simulink model "px4demo_rgbled"  (R2014b)
settings: Solver=ode3  SolverMode=SingleTasking  StartTime=0.0  StopTime=10.0  FixedStep=1/250  RelTol=1e-3
PostLoadFcn:
  | Ts = 1/250;
undefined symbols (not defined in the file): RGBLED_COLOR_ENUM, RGBLED_MODE_ENUM
libraries: pixhawk_sllib x1
settings Model: Creator=skuznick  LastModifiedBy=skuznick
settings OptimizationCC: InlineParams=on  OptimizeModelRefInitCode=on  LifeSpan=1  MaxStackSize=64
settings HardwareCC: ProdLargestAtomicInteger=Long  ProdLargestAtomicFloat=Double  ProdEndianess=LittleEndian  ProdHWDeviceType=ARM Compatible->ARM Cortex
settings RTWCC: SystemTargetFile=ert.tlc  TLCOptions=-aInlineSetEventsForThisBaseRateFcn=TLC_FALSE -aSuppressMultiTaskScheduler=TLC_FALSE  TemplateMakefile=ert_default_tmf  Description=Embedded Coder  GenerateReport=on  ProcessScript=ert_make_rtw_hook  Toolchain=Pixhawk Toolchain  IncludeHyperlinkInReport=on  LaunchReport=on  GenerateTraceReport=on  GenerateCodeMetricsReport=on
settings CodeAppCC: IgnoreCustomStorageClasses=off

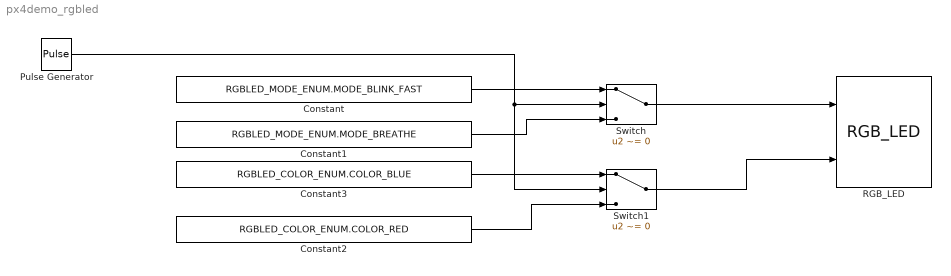
== system px4demo_rgbled ==
  Constant : Constant  Value=RGBLED_MODE_ENUM.MODE_BLINK_FAST  OutDataTypeStr=Enum: RGBLED_MODE_ENUM
  Constant1 : Constant  Value=RGBLED_MODE_ENUM.MODE_BREATHE  OutDataTypeStr=Enum: RGBLED_MODE_ENUM
  Constant2 : Constant  Value=RGBLED_COLOR_ENUM.COLOR_RED  OutDataTypeStr=Enum: RGBLED_COLOR_ENUM
  Constant3 : Constant  Value=RGBLED_COLOR_ENUM.COLOR_BLUE  OutDataTypeStr=Enum: RGBLED_COLOR_ENUM
  Pulse Generator : DiscretePulseGenerator  PulseType=Time based  PulseWidth=50
  RGB_LED : pixhawk_sllib/RGB_LED
  Switch : Switch  Criteria=u2 ~= 0  Threshold=1500
  Switch1 : Switch  Criteria=u2 ~= 0  Threshold=1500
  wires:
  Switch/1 -> RGB_LED/1
  Switch1/1 -> RGB_LED/2
  Constant/1 -> Switch/1
  Constant1/1 -> Switch/3
  Constant3/1 -> Switch1/1
  Constant2/1 -> Switch1/3
  Pulse Generator/1 -> Switch1/2, Switch/2
